simulink model "scdcstr"  (Simulink 7.6)
settings: Solver=ode45  StartTime=0  StopTime=60  MaxStep=0.2  RelTol=1e-3
model workspace (MATLAB code in the model file):
  | %Model constants
  | k0                = 34930800;
  | DeltaER       = 5963.6;
  | DeltaH         = -11.92;
  | UA               = 0.3;
  | FV_plus_UA = 1.3;
  | 
  | %Fixed IC
  | Concentration0 = 2;
  | FeedCon0         = 10;
  | FeedTemp0       = 295;
  | 
  | %Derived IC
  | tmpVal = FeedCon0/Concentration0-1;
  | ReactorTemp0 = -DeltaER/log(tmpVal/k0);
  | CoolantTemp0 = (ReactorTemp0*(FV_plus_UA)+tmpVal*Concentration0*DeltaH-FeedTemp0)/UA;
libraries: simulink x3, slctrlblks x1, simulink_extras x1
settings Model: Creator=The MathWorks Inc.  BufferReuse=off
settings DataIOCC: InitialState=[311.267; 8.5695]  SignalLoggingName=logsOut
settings OptimizationCC: BlockReduction=off  BooleanDataType=off  InlineParams=on  InlineInvariantSignals=on  BufferReuse=off  InitFltsAndDblsToZero=on
settings DebuggingCC: SaveWithParameterizedLinksMsg=none  CheckExecutionContextPreStartOutputMsg=on  CheckExecutionContextRuntimeOutputMsg=on  SignalResolutionControl=TryResolveAllWithWarning  SolverPrmCheckMsg=none  MultiTaskDSMMsg=warning  MultiTaskCondExecSysMsg=none  StrictBusMsg=None
settings HardwareCC: TargetUnknown=on
settings RTWCC: IncludeERTFirstTime=on
settings GRTTargetCC: TargetFcnLib=ansi_tfl_tmw.mat

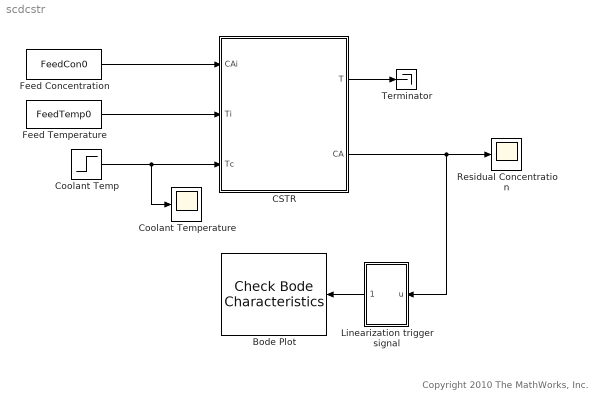
== system scdcstr ==
  note: Copyright 2010 The MathWorks, Inc.
  Bode Plot : slctrlblks/Model Verification/Check Bode  Characteristics  InstantiateOnLoad=on  DialogController=checkpack.createCheckDlg  DialogControllerArgs=DataTag0  SystemSampleTime=-1  LinearizationIOs={'/Coolant Temp', 1, 'in', 'off';'/CSTR', 2, 'out', 'off'}  LinearizeAt=ExternalTrigger  SnapshotTimes=[0]  TriggerType=rising  ZeroCross=off  SampleTime=auto  RateConversionMethod=zoh  PreWarpFreq=10  UseExactDelayModel=off  UseFullBlockNameLabels=off  UseBusSignalLabels=off  enabled=on  stopWhenAssertionFail=off  export=off  ViewDlgPos=[127 134 510 390]  OpenViewOnLoad=off  LaunchViewOnOpen=off  FrequencyUnits=rad/sec  MagnitudeUnits=dB  PhaseUnits=deg  EnableUpperBound=off  UpperBoundFrequencies=[]  UpperBoundMagnitudes=[]  EnableLowerBound=off  LowerBoundFrequencies=[]  LowerBoundMagnitudes=[]
      settings: SaveToWorkspace=on  SaveName=LinearReactor
  CSTR : Subsystem
  Coolant Temp : Step  Time=20  Before=CoolantTemp0  After=CoolantTemp0*(1-0.05)  SampleTime=0
  Coolant Temperature : Scope
      settings: TimeRange=60  YMin=295  YMax=320  SaveName=ScopeData2
  Feed Concentration : Constant  Value=FeedCon0
  Feed Temperature : Constant  Value=FeedTemp0
  Linearization trigger signal : Subsystem
  Residual Concentration : Scope
      settings: TimeRange=60  YMin=0  YMax=10
  Terminator : Terminator
  wires:
  CSTR/2(CA) -> Residual Concentration/1, Linearization trigger signal/1(u)
  Feed Concentration/1 -> CSTR/1(CAi)
  Feed Temperature/1 -> CSTR/2(Ti)
  Coolant Temp/1 -> CSTR/3(Tc), Coolant Temperature/1
  Linearization trigger signal/1(trigger) -> Bode Plot/1
  CSTR/1(T) -> Terminator/1

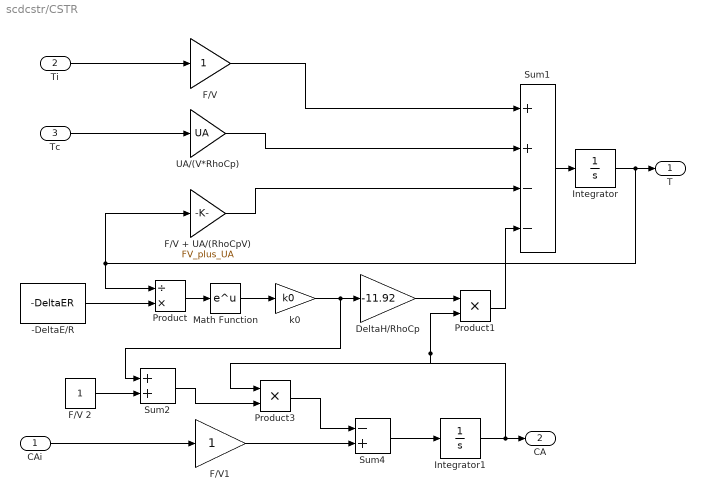
== system scdcstr/CSTR ==
  CAi : Inport
  Ti : Inport  Port=2
  Tc : Inport  Port=3
  -DeltaE/R : Constant  Value=-DeltaER
  DeltaH/RhoCp : Gain  Gain=-11.92  SaturateOnIntegerOverflow=on  OutDataTypeStr=Inherit: Same as input  ParamDataTypeStr=Inherit: Same as input
  F/V : Gain  SaturateOnIntegerOverflow=on  OutDataTypeStr=Inherit: Same as input  ParamDataTypeStr=Inherit: Same as input
  F/V + UA/(RhoCpV) : Gain  Gain=FV_plus_UA  SaturateOnIntegerOverflow=on  OutDataTypeStr=Inherit: Same as input  ParamDataTypeStr=Inherit: Same as input
  F/V 2 : Constant
  F/V1 : Gain  SaturateOnIntegerOverflow=on  OutDataTypeStr=Inherit: Same as input  ParamDataTypeStr=Inherit: Same as input
  Integrator : Integrator  InitialCondition=ReactorTemp0  LimitOutput=on  LowerSaturationLimit=0
  Integrator1 : Integrator  InitialCondition=Concentration0  LimitOutput=on  LowerSaturationLimit=0
  Math Function : Math  SaturateOnIntegerOverflow=on
  Product : Product  Inputs=/*  SaturateOnIntegerOverflow=on  RndMeth=Zero  InputSameDT=on  OutDataTypeStr=Inherit: Same as first input
  Product1 : Product  SaturateOnIntegerOverflow=on  RndMeth=Zero  InputSameDT=on  OutDataTypeStr=Inherit: Same as first input
  Product3 : Product  SaturateOnIntegerOverflow=on  RndMeth=Zero  InputSameDT=on  OutDataTypeStr=Inherit: Same as first input
  Sum1 : Sum  Inputs=++--  SaturateOnIntegerOverflow=on  InputSameDT=on  OutDataTypeStr=Inherit: Same as first input
  Sum2 : Sum  SaturateOnIntegerOverflow=on  InputSameDT=on  OutDataTypeStr=Inherit: Same as first input
  Sum4 : Sum  Inputs=-+  SaturateOnIntegerOverflow=on  InputSameDT=on  OutDataTypeStr=Inherit: Same as first input
  UA/(V*RhoCp) : Gain  Gain=UA  SaturateOnIntegerOverflow=on  OutDataTypeStr=Inherit: Same as input  ParamDataTypeStr=Inherit: Same as input
  k0 : Gain  Gain=k0  SaturateOnIntegerOverflow=on  OutDataTypeStr=Inherit: Same as input  ParamDataTypeStr=Inherit: Same as input
  T : Outport
  CA : Outport  Port=2
  wires:
  F/V/1 -> Sum1/1
  Sum1/1 -> Integrator/1
  Integrator/1 -> Product/1, F/V + UA/(RhoCpV)/1, T/1
  UA/(V*RhoCp)/1 -> Sum1/2
  F/V + UA/(RhoCpV)/1 -> Sum1/3
  Product/1 -> Math Function/1
  Math Function/1 -> k0/1
  DeltaH/RhoCp/1 -> Product1/1
  Product1/1 -> Sum1/4
  k0/1 -> DeltaH/RhoCp/1, Sum2/1
  -DeltaE/R/1 -> Product/2
  Product3/1 -> Sum4/1
  Sum4/1 -> Integrator1/1
  Integrator1/1 -> Product3/1, Product1/2, CA/1
  F/V 2/1 -> Sum2/2
  F/V1/1 -> Sum4/2
  Ti/1 -> F/V/1
  CAi/1 -> F/V1/1
  Tc/1 -> UA/(V*RhoCp)/1
  Sum2/1 -> Product3/2

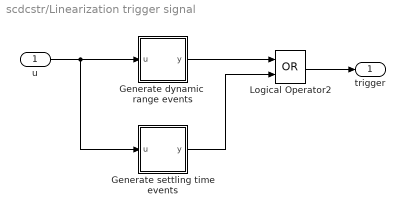
== system scdcstr/Linearization trigger signal ==
  u : Inport
  Generate dynamic  range events : Subsystem  mask(Dynamic Range Trigger Generator){UB=5.5, LB=4.5}
      mask prompts: UB "Signal upper bound"; LB "Signal lower bound"
      mask help: Generates trigger events when a signal enters and exits a dynamic range. When the signal enters the dynamic range a rising edge event is fired, a falling edge event is fired when the signal leaves the dynamic range.
      mask init:
      | if length(UB) ~= length(LB)
      | 	error('The upper and lower bound settling time values must be the same.')
      | end
      mask Help:
      | <p>
      | The dynamic range trigger generator outputs trigger events when a signal enters and exits a
      | dynamic range. A rising edge event is fired when the signal enters the dynamic range specified
      | by the block parameters. A falling edge event is fired when the signal exits the dynamic range
      | specified by the block parameters.
      | </p>
      | 
      | <p>
      | Mask variables:
      | </p>
      | <ul>
      | <li> Signal upper bound - Upper limits for the signal dynamic range.  This is a vector. </li>
      | <li> Signal lower bound - Lower limits for the signal dynamic range.  This is a vector. </li>
      | </ul>
  Generate settling time events : Subsystem  mask(Settling Time Trigger Generator){ub=[2.5 9.5], lb=[1.5 8.5], interval=5}
      mask prompts: ub "Settling Time Upper Bounds"; lb "Settling Time Lower Bound"; interval "Settling Interval (sec.)"
      mask help: Generates trigger events for when a system comes to be within settling intervals specified in the block mask.
      mask init:
      | if length(ub) ~= length(lb)
      | 	error('The upper and lower bound settling time values must be the same.')
      | end
      mask Help:
      | <p>
      | The settling time trigger generator outputs trigger events for when a system comes to be within settling intervals specified in the block mask.
      | </p>
      | 
      | <p>
      | Mask variables:
      | </p>
      | <ul>
      | <li> Settling Time Upper Bounds - Upper limits for system settling.  This is a vector. </li>
      | <li> Settling Time Lower Bounds - Lower limits for system settling.  This is a vector. </li>
      | <li> Settling Interval - Time that a signal must be inside the settling region before a rising edge trigger is output from the block. </li>
      | </ul>
  Logical Operator2 : Logic  Operator=OR  AllPortsSameDT=off  OutDataTypeStr=boolean
  trigger : Outport
  wires:
  u/1 -> Generate settling time events/1(u), Generate dynamic  range events/1(u)
  Generate dynamic  range events/1(y) -> Logical Operator2/1
  Generate settling time events/1(y) -> Logical Operator2/2
  Logical Operator2/1 -> trigger/1

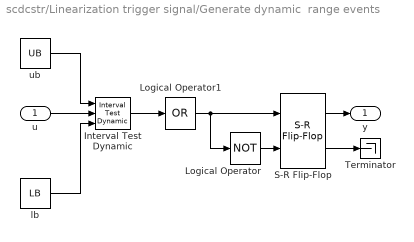
== system scdcstr/Linearization trigger signal/Generate dynamic  range events ==
  u : Inport
  Interval Test Dynamic : simulink/Logic and Bit Operations/Interval Test Dynamic  SystemSampleTime=-1  IntervalClosedRight=on  IntervalClosedLeft=on  LogicOutDataTypeMode=boolean
  Logical Operator : Logic  Operator=NOT  AllPortsSameDT=off  OutDataTypeStr=boolean
  Logical Operator1 : Logic  Operator=OR  Inputs=1  AllPortsSameDT=off  OutDataTypeStr=boolean
  S-R Flip-Flop : simulink_extras/Flip Flops/S-R Flip-Flop  SystemSampleTime=-1  initial_condition=0
  Terminator : Terminator
  lb : Constant  Value=LB
  ub : Constant  Value=UB
  y : Outport
  wires:
  Logical Operator/1 -> S-R Flip-Flop/2
  S-R Flip-Flop/2 -> Terminator/1
  Interval Test Dynamic/1 -> Logical Operator1/1
  ub/1 -> Interval Test Dynamic/1
  lb/1 -> Interval Test Dynamic/3
  Logical Operator1/1 -> S-R Flip-Flop/1, Logical Operator/1
  u/1 -> Interval Test Dynamic/2
  S-R Flip-Flop/1 -> y/1

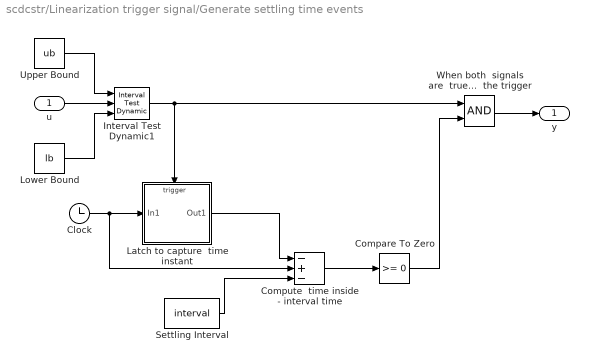
== system scdcstr/Linearization trigger signal/Generate settling time events ==
  u : Inport
  Clock : Clock
      settings: Decimation=10
  Compare To Zero : simulink/Logic and Bit Operations/Compare To Zero  SystemSampleTime=-1  relop=>=  LogicOutDataTypeMode=uint8  ZeroCross=off
  "Compute  time inside - interval time  " : Sum  Inputs=-+-  OutDataTypeStr=double
  Interval Test Dynamic1 : simulink/Logic and Bit Operations/Interval Test Dynamic  SystemSampleTime=-1  IntervalClosedRight=on  IntervalClosedLeft=on  LogicOutDataTypeMode=uint8
  Latch to capture  time instant : Subsystem  TreatAsAtomicUnit=on
  Lower Bound : Constant  Value=lb
  Settling Interval : Constant  Value=interval
  Upper Bound : Constant  Value=ub
  "When both  signals are  true throw  the trigger " : Logic  AllPortsSameDT=off  OutDataTypeStr=boolean
  y : Outport
  wires:
  Interval Test Dynamic1/1 -> "When both  signals are  true throw  the trigger "/1, Latch to capture  time instant/Trigger
  Clock/1 -> "Compute  time inside - interval time  "/2, Latch to capture  time instant/1(In1)
  Compare To Zero/1 -> "When both  signals are  true throw  the trigger "/2
  Lower Bound/1 -> Interval Test Dynamic1/3
  u/1 -> Interval Test Dynamic1/2
  Upper Bound/1 -> Interval Test Dynamic1/1
  "When both  signals are  true throw  the trigger "/1 -> y/1
  Latch to capture  time instant/1(Out1) -> "Compute  time inside - interval time  "/1
  "Compute  time inside - interval time  "/1 -> Compare To Zero/1
  Settling Interval/1 -> "Compute  time inside - interval time  "/3

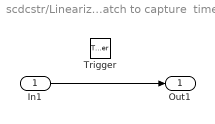
== system scdcstr/Linearization trigger signal/Generate settling time events/Latch to capture  time instant ==
  In1 : Inport
  Trigger : TriggerPort  OutputDataType=double  ZeroCross=off
  Out1 : Outport  InitialOutput=0
  wires:
  In1/1 -> Out1/1
